simulink model "MuscleModel_ThelenRigid"  (R2024b)
settings: Solver=VariableStepAuto  StartTime=0.0  StopTime=10.0  RelTol=1e-3
undefined symbols (not defined in the file or in its folder): alpha0, FM0, LM0, LTs
settings Model: Creator=jakub  LastModifiedBy=jakub

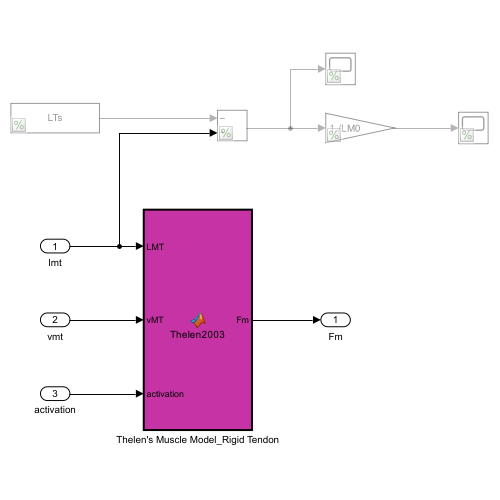
[thumbnail: Simulink's stored preview of the top-level diagram]
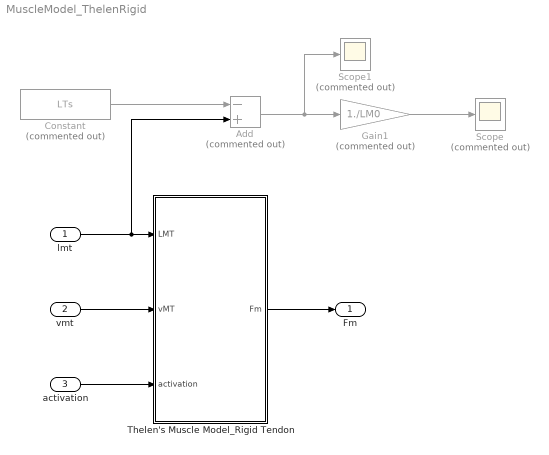
== system MuscleModel_ThelenRigid ==
  lmt : Inport  OutDataTypeStr=double  Unit=m  PortDimensions=[8 1]  SampleTime=0
  vmt : Inport  Port=2  OutDataTypeStr=double  Unit=m/s  PortDimensions=[8 1]  SampleTime=0
  activation : Inport  Port=3  OutDataTypeStr=double  PortDimensions=[8 1]  SampleTime=0
  Add : Sum  Commented=on  Inputs=-+
  Constant : Constant  Commented=on  Value=LTs
  Gain1 : Gain  Commented=on  Gain=1./LM0
  Scope : Scope  Commented=on
  Scope1 : Scope  Commented=on
  Thelen's Muscle Model_Rigid Tendon : MATLAB Function  TreatAsAtomicUnit=on
  Fm : Outport  OutDataTypeStr=double  Unit=N  PortDimensions=[8 1]
  wires:
  lmt/1 -> Add/2, Thelen's Muscle Model_Rigid Tendon/1(LMT)
  Thelen's Muscle Model_Rigid Tendon/1(Fm) -> Fm/1
  activation/1 -> Thelen's Muscle Model_Rigid Tendon/3(activation)
  Constant/1 -> Add/1
  Gain1/1 -> Scope/1
  Add/1 -> Scope1/1, Gain1/1
  vmt/1 -> Thelen's Muscle Model_Rigid Tendon/2(vMT)

== matlab function MuscleModel_ThelenRigid/Thelen's Muscle Model_Rigid Tendon ==
  data: LMT input double size=[8 1]; vMT input double size=[8 1]; Fm output double size=[8 1]; activation input double size=[8 1]; LM0 parameter double size=[8 1]; LTs parameter double size=[8 1]; FM0 parameter double size=[8 1]; alpha0 parameter
function Fm  = Thelen2003(LMT, vMT, activation, LM0, LTs, FM0, alpha0)

    % Muscle constants
        epsM0 = 0.6;            % passive muscle strain due to maximum isometric force
        kPE = 4;                % an exponential shape factor for the passive force-length relationship
        gamma = 0.5;            % a shape factor for the Gaussian active force-length relationship
        Af = 0.3;               % a shape factor for the force-velocity relationship
        fMlen = 1.4;            % maximum normalized muscle force achievable when the fiber is lengthening
        VMmax = 10;


    Fm = zeros(numel(activation),1);
    
    for k = 1:numel(LM0)
        Lmt = LMT(k);
        Lt = LTs(k);
        Lm0 = LM0(k);
        Fm0 = FM0(k);
        vmt = vMT(k);
        a = activation(k);
        alpha = alpha0(k);

    %% Muscle length and velocity
        Lm = (Lmt - Lt)/cos(alpha);
        Vm = vmt*cos(alpha);

        lm = Lm/Lm0;

    %% Force of the (contractile element) - ACTIVE FORCE
        fl = exp(-(lm-1)^2/gamma);
        if fl < 0.1
            fl = 0.1;
        end

    %% Force of the muscle parallel element - PASSIVE FORCE
        fpe = (exp(kPE*(lm - 1)/epsM0) - 1) / (exp(kPE) - 1);
        if fpe < 0
            fpe = 0;
        end

    %% Force of the contractile element - Force-velocity relation
        vmmax = VMmax*Lm0;

        if Vm <= 0
            fvm = Af*(4*Vm + vmmax*(3*a + 1)) / (-4*Vm + vmmax*Af*(3*a + 1));
        else
            fvm = (Af*vmmax*(3*a*fMlen - 3*a + fMlen - 1) + 8*Vm*fMlen*(Af + 1)) / (Af*vmmax*(3*a*fMlen - 3*a + fMlen - 1) + 8*Vm*(Af + 1));
        end


    %% Muscle Force
        Fm(k) = Fm0*(a*fl*fvm + fpe)*cos(alpha);
    end
        


end
